simulink model "ModelCurrentState"  (R2024b)
settings: Solver=VariableStepAuto  StartTime=0.0  StopTime=StopTime  MaxStep=0.001  RelTol=1e-3
model workspace: external: MAT-File 3DModelInputs.mat (data not in the file)
undefined symbols (not defined in the file): GripStrength, KillswitchFinalValue, KillswitchInitialValue, KillswitchStepTime, LeftLowerArmLength, PlaneTilt, RightLowerArmLength, UpperTorsoLength, X, Y, Z
libraries: nesl_utility x408, sm_lib x139, matrix_library x11, simulink x1
(part 8 of 14)

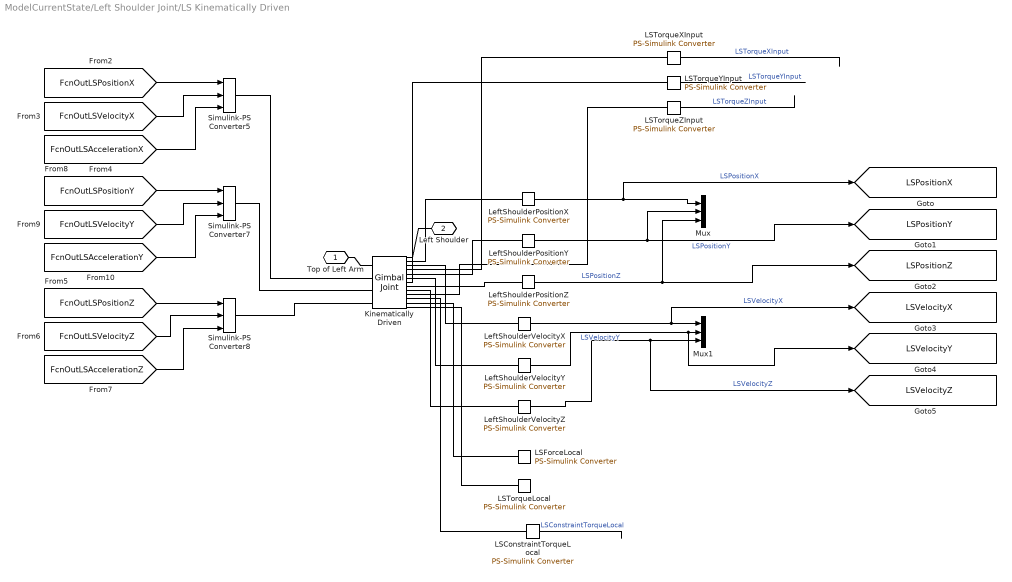
== system ModelCurrentState/Left Shoulder Joint/LS Kinematically Driven ==
  Kinematically Driven : sm_lib/Joints/Gimbal Joint  JointMode=Normal  CompositeWrenchDir=BaseOnFollower  CompositeWrenchFrame=FollowerFrame  SenseConstraintForce=off  SenseConstraintTorque=on  SenseTotalForce=on  SenseTotalTorque=on  RxPositionTargetSpecify=off  RxPositionTargetPriority=Low  RxPositionTargetValue=LSStartPositionX  RxPositionTargetValueUnits=deg  RxVelocityTargetSpecify=off  RxVelocityTargetPriority=Low  RxVelocityTargetValue=LSStartVelocityX  RxVelocityTargetValueUnits=deg/s  RxEquilibriumPosition=120  RxEquilibriumPositionUnits=deg  RxSpringStiffness=0  RxSpringStiffnessUnits=N*m/deg  RxDampingCoefficient=0  RxDampingCoefficientUnits=N*m/(deg/s)  RxLowerLimitSpecify=off  RxLowerLimitBound=-80  RxLowerLimitBoundUnits=deg  RxLowerLimitStiffness=100  RxLowerLimitStiffnessUnits=N*m/deg  RxLowerLimitDamping=10  RxLowerLimitDampingUnits=N*m/(deg/s)  RxLowerLimitTransitionRegionWidth=0.1  RxLowerLimitTransitionRegionWidthUnits=deg  RxUpperLimitSpecify=off  RxUpperLimitBound=80  RxUpperLimitBoundUnits=deg  RxUpperLimitStiffness=100  RxUpperLimitStiffnessUnits=N*m/deg  RxUpperLimitDamping=10  RxUpperLimitDampingUnits=N*m/(deg/s)  RxUpperLimitTransitionRegionWidth=0.1  RxUpperLimitTransitionRegionWidthUnits=deg  RxTorqueActuationMode=ComputedTorque  RxMotionActuationMode=InputMotion  RxSensePosition=on  RxSenseVelocity=on  RxSenseAcceleration=off  RxSenseTorqueForce=on  RxSenseLowerLimitTorqueForce=off  RxSenseUpperLimitTorqueForce=off  RyPositionTargetSpecify=off  RyPositionTargetPriority=Low  RyPositionTargetValue=LSStartPositionY  RyPositionTargetValueUnits=deg  RyVelocityTargetSpecify=off  RyVelocityTargetPriority=Low  RyVelocityTargetValue=LSStartVelocityY  RyVelocityTargetValueUnits=deg/s  RyEquilibriumPosition=0  RyEquilibriumPositionUnits=deg  RySpringStiffness=0  RySpringStiffnessUnits=N*m/deg  RyDampingCoefficient=0  RyDampingCoefficientUnits=N*m/(deg/s)  RyLowerLimitSpecify=off  RyLowerLimitBound=-80  RyLowerLimitBoundUnits=deg  RyLowerLimitStiffness=100  RyLowerLimitStiffnessUnits=N*m/deg  RyLowerLimitDamping=10  RyLowerLimitDampingUnits=N*m/(deg/s)  RyLowerLimitTransitionRegionWidth=0.1  RyLowerLimitTransitionRegionWidthUnits=deg  RyUpperLimitSpecify=off  RyUpperLimitBound=80  RyUpperLimitBoundUnits=deg  RyUpperLimitStiffness=100  RyUpperLimitStiffnessUnits=N*m/deg  RyUpperLimitDamping=10  RyUpperLimitDampingUnits=N*m/(deg/s)  RyUpperLimitTransitionRegionWidth=0.1  RyUpperLimitTransitionRegionWidthUnits=deg  RyTorqueActuationMode=ComputedTorque  RyMotionActuationMode=InputMotion  RySensePosition=on  RySenseVelocity=on  RySenseAcceleration=off  RySenseTorqueForce=on  RySenseLowerLimitTorqueForce=off  RySenseUpperLimitTorqueForce=off  RzPositionTargetSpecify=off  RzPositionTargetPriority=Low  RzPositionTargetValue=LSStartPositionZ  RzPositionTargetValueUnits=deg  RzVelocityTargetSpecify=off  RzVelocityTargetPriority=Low  RzVelocityTargetValue=LSStartVelocityZ  RzVelocityTargetValueUnits=deg/s  RzEquilibriumPosition=0  RzEquilibriumPositionUnits=deg  RzSpringStiffness=0  RzSpringStiffnessUnits=N*m/deg  RzDampingCoefficient=0  RzDampingCoefficientUnits=N*m/(deg/s)  RzLowerLimitSpecify=off  RzLowerLimitBound=-180  RzLowerLimitBoundUnits=deg  RzLowerLimitStiffness=100  RzLowerLimitStiffnessUnits=N*m/deg  RzLowerLimitDamping=10  RzLowerLimitDampingUnits=N*m/(deg/s)  RzLowerLimitTransitionRegionWidth=0.1  RzLowerLimitTransitionRegionWidthUnits=deg  RzUpperLimitSpecify=off  RzUpperLimitBound=-95  RzUpperLimitBoundUnits=deg  RzUpperLimitStiffness=100  RzUpperLimitStiffnessUnits=N*m/deg  RzUpperLimitDamping=10  RzUpperLimitDampingUnits=N*m/(deg/s)  RzUpperLimitTransitionRegionWidth=0.1  RzUpperLimitTransitionRegionWidthUnits=deg  RzTorqueActuationMode=ComputedTorque  RzMotionActuationMode=InputMotion  RzSensePosition=on  RzSenseVelocity=on  RzSenseAcceleration=off  RzSenseTorqueForce=on  RzSenseLowerLimitTorqueForce=off  RzSenseUpperLimitTorqueForce=off
  LSConstraintTorqueLocal : nesl_utility/PS-Simulink Converter  PhysicalDomain=network_engine_domain  SubClassName=ps_output  LeftPortType=input  RightPortType=output  PseudoPeriodic=off  Frequencies=[]  VectorFormat=1-D array  Unit=inherit  AffineConversion=off
  LSForceLocal : nesl_utility/PS-Simulink Converter  PhysicalDomain=network_engine_domain  SubClassName=ps_output  LeftPortType=input  RightPortType=output  PseudoPeriodic=off  Frequencies=[]  VectorFormat=1-D array  Unit=inherit  AffineConversion=off
  LSTorqueLocal : nesl_utility/PS-Simulink Converter  PhysicalDomain=network_engine_domain  SubClassName=ps_output  LeftPortType=input  RightPortType=output  PseudoPeriodic=off  Frequencies=[]  VectorFormat=1-D array  Unit=inherit  AffineConversion=off
  LSTorqueXInput : nesl_utility/PS-Simulink Converter  PhysicalDomain=network_engine_domain  SubClassName=ps_output  LeftPortType=input  RightPortType=output  PseudoPeriodic=off  Frequencies=[]  VectorFormat=1-D array  Unit=inherit  AffineConversion=off
  LSTorqueYInput : nesl_utility/PS-Simulink Converter  PhysicalDomain=network_engine_domain  SubClassName=ps_output  LeftPortType=input  RightPortType=output  PseudoPeriodic=off  Frequencies=[]  VectorFormat=1-D array  Unit=inherit  AffineConversion=off
  LSTorqueZInput : nesl_utility/PS-Simulink Converter  PhysicalDomain=network_engine_domain  SubClassName=ps_output  LeftPortType=input  RightPortType=output  PseudoPeriodic=off  Frequencies=[]  VectorFormat=1-D array  Unit=inherit  AffineConversion=off
  LeftShoulderPositionX : nesl_utility/PS-Simulink Converter  PhysicalDomain=network_engine_domain  SubClassName=ps_output  LeftPortType=input  RightPortType=output  PseudoPeriodic=off  Frequencies=[]  VectorFormat=1-D array  Unit=deg  AffineConversion=off
  LeftShoulderPositionY : nesl_utility/PS-Simulink Converter  PhysicalDomain=network_engine_domain  SubClassName=ps_output  LeftPortType=input  RightPortType=output  PseudoPeriodic=off  Frequencies=[]  VectorFormat=1-D array  Unit=deg  AffineConversion=off
  LeftShoulderPositionZ : nesl_utility/PS-Simulink Converter  PhysicalDomain=network_engine_domain  SubClassName=ps_output  LeftPortType=input  RightPortType=output  PseudoPeriodic=off  Frequencies=[]  VectorFormat=1-D array  Unit=deg  AffineConversion=off
  LeftShoulderVelocityX : nesl_utility/PS-Simulink Converter  PhysicalDomain=network_engine_domain  SubClassName=ps_output  LeftPortType=input  RightPortType=output  PseudoPeriodic=off  Frequencies=[]  VectorFormat=1-D array  Unit=deg/s  AffineConversion=off
  LeftShoulderVelocityY : nesl_utility/PS-Simulink Converter  PhysicalDomain=network_engine_domain  SubClassName=ps_output  LeftPortType=input  RightPortType=output  PseudoPeriodic=off  Frequencies=[]  VectorFormat=1-D array  Unit=deg/s  AffineConversion=off
  LeftShoulderVelocityZ : nesl_utility/PS-Simulink Converter  PhysicalDomain=network_engine_domain  SubClassName=ps_output  LeftPortType=input  RightPortType=output  PseudoPeriodic=off  Frequencies=[]  VectorFormat=1-D array  Unit=deg/s  AffineConversion=off
  Mux : Mux  Inputs=3
  Mux1 : Mux  Inputs=3
  Simulink-PS Converter5 : nesl_utility/Simulink-PS Converter  PhysicalDomain=network_engine_domain  SubClassName=ps_input  LeftPortType=input  RightPortType=output  PseudoPeriodic=off  Frequencies=[]  NoiseDistribution=none  NoiseParameters=[]  Unit=deg  AffineConversion=off  FilteringAndDerivatives=provide  SimscapeFilterOrder=1  InputFilterTimeConstant=0.001  UdotUserProvided=2
  Simulink-PS Converter7 : nesl_utility/Simulink-PS Converter  PhysicalDomain=network_engine_domain  SubClassName=ps_input  LeftPortType=input  RightPortType=output  PseudoPeriodic=off  Frequencies=[]  NoiseDistribution=none  NoiseParameters=[]  Unit=deg  AffineConversion=off  FilteringAndDerivatives=provide  SimscapeFilterOrder=1  InputFilterTimeConstant=0.001  UdotUserProvided=2
  Simulink-PS Converter8 : nesl_utility/Simulink-PS Converter  PhysicalDomain=network_engine_domain  SubClassName=ps_input  LeftPortType=input  RightPortType=output  PseudoPeriodic=off  Frequencies=[]  NoiseDistribution=none  NoiseParameters=[]  Unit=deg  AffineConversion=off  FilteringAndDerivatives=provide  SimscapeFilterOrder=1  InputFilterTimeConstant=0.001  UdotUserProvided=2
  Top of Left Arm : PMIOPort  Side=Left
  Left Shoulder : PMIOPort  Port=2  Side=Right
  tag scope: LSPositionX=global, LSPositionY=global, LSPositionZ=global, LSVelocityX=global, LSVelocityY=global, LSVelocityZ=global
  wires:
  [FcnOutLSPositionX] -> Simulink-PS Converter5/1
  [FcnOutLSPositionZ] -> Simulink-PS Converter8/1
  [FcnOutLSPositionY] -> Simulink-PS Converter7/1
  [FcnOutLSAccelerationZ] -> Simulink-PS Converter8/3
  [FcnOutLSAccelerationX] -> Simulink-PS Converter5/3
  [FcnOutLSAccelerationY] -> Simulink-PS Converter7/3
  [FcnOutLSVelocityY] -> Simulink-PS Converter7/2
  [FcnOutLSVelocityX] -> Simulink-PS Converter5/2
  [FcnOutLSVelocityZ] -> Simulink-PS Converter8/2
  LeftShoulderPositionY/1 -> [LSPositionY], Mux/2  "LSPositionY"
  LeftShoulderVelocityY/1 -> [LSVelocityY], Mux1/2  "LSVelocityY"
  LeftShoulderPositionZ/1 -> Mux/3, [LSPositionZ]  "LSPositionZ"
  LeftShoulderVelocityX/1 -> [LSVelocityX], Mux1/1  "LSVelocityX"
  LeftShoulderPositionX/1 -> [LSPositionX], Mux/1  "LSPositionX"
  LeftShoulderVelocityZ/1 -> [LSVelocityZ], Mux1/3  "LSVelocityZ"
  LSConstraintTorqueLocal/1 -> ?  "LSConstraintTorqueLocal"
  LSTorqueYInput/1 -> ?  "LSTorqueYInput"
  LSTorqueXInput/1 -> ?  "LSTorqueXInput"
  LSTorqueZInput/1 -> ?  "LSTorqueZInput"
  connections:
  Kinematically Driven/LConn1 -- Top of Left Arm/RConn1
  Simulink-PS Converter5/RConn1 -- Kinematically Driven/LConn2
  Simulink-PS Converter7/RConn1 -- Kinematically Driven/LConn3
  Simulink-PS Converter8/RConn1 -- Kinematically Driven/LConn4
  Left Shoulder/RConn1 -- Kinematically Driven/RConn1
  Kinematically Driven/RConn2 -- LeftShoulderPositionX/LConn1
  Kinematically Driven/RConn5 -- LeftShoulderPositionY/LConn1
  Kinematically Driven/RConn8 -- LeftShoulderPositionZ/LConn1
  Kinematically Driven/RConn3 -- LeftShoulderVelocityX/LConn1
  Kinematically Driven/RConn6 -- LeftShoulderVelocityY/LConn1
  Kinematically Driven/RConn9 -- LeftShoulderVelocityZ/LConn1
  LSForceLocal/LConn1 -- Kinematically Driven/RConn12
  LSTorqueLocal/LConn1 -- Kinematically Driven/RConn13
  Kinematically Driven/RConn11 -- LSConstraintTorqueLocal/LConn1
  LSTorqueXInput/LConn1 -- Kinematically Driven/RConn4
  LSTorqueYInput/LConn1 -- Kinematically Driven/RConn7
  LSTorqueZInput/LConn1 -- Kinematically Driven/RConn10

== system ModelCurrentState/Left Shoulder Joint/LS Kinetically Driven ==
  Kinetically Driven : sm_lib/Joints/Gimbal Joint  JointMode=Normal  CompositeWrenchDir=BaseOnFollower  CompositeWrenchFrame=FollowerFrame  SenseConstraintForce=off  SenseConstraintTorque=on  SenseTotalForce=on  SenseTotalTorque=on  RxPositionTargetSpecify=on  RxPositionTargetPriority=Low  RxPositionTargetValue=LSStartPositionX  RxPositionTargetValueUnits=deg  RxVelocityTargetSpecify=on  RxVelocityTargetPriority=Low  RxVelocityTargetValue=LSStartVelocityX  RxVelocityTargetValueUnits=deg/s  RxEquilibriumPosition=120  RxEquilibriumPositionUnits=deg  RxSpringStiffness=0  RxSpringStiffnessUnits=N*m/deg  RxDampingCoefficient=0  RxDampingCoefficientUnits=N*m/(deg/s)  RxLowerLimitSpecify=off  RxLowerLimitBound=-80  RxLowerLimitBoundUnits=deg  RxLowerLimitStiffness=100  RxLowerLimitStiffnessUnits=N*m/deg  RxLowerLimitDamping=10  RxLowerLimitDampingUnits=N*m/(deg/s)  RxLowerLimitTransitionRegionWidth=0.1  RxLowerLimitTransitionRegionWidthUnits=deg  RxUpperLimitSpecify=off  RxUpperLimitBound=80  RxUpperLimitBoundUnits=deg  RxUpperLimitStiffness=100  RxUpperLimitStiffnessUnits=N*m/deg  RxUpperLimitDamping=10  RxUpperLimitDampingUnits=N*m/(deg/s)  RxUpperLimitTransitionRegionWidth=0.1  RxUpperLimitTransitionRegionWidthUnits=deg  RxTorqueActuationMode=InputTorque  RxMotionActuationMode=ComputedMotion  RxSensePosition=on  RxSenseVelocity=on  RxSenseAcceleration=off  RxSenseTorqueForce=on  RxSenseLowerLimitTorqueForce=off  RxSenseUpperLimitTorqueForce=off  RyPositionTargetSpecify=on  RyPositionTargetPriority=Low  RyPositionTargetValue=LSStartPositionY  RyPositionTargetValueUnits=deg  RyVelocityTargetSpecify=on  RyVelocityTargetPriority=Low  RyVelocityTargetValue=LSStartVelocityY  RyVelocityTargetValueUnits=deg/s  RyEquilibriumPosition=0  RyEquilibriumPositionUnits=deg  RySpringStiffness=0  RySpringStiffnessUnits=N*m/deg  RyDampingCoefficient=0  RyDampingCoefficientUnits=N*m/(deg/s)  RyLowerLimitSpecify=off  RyLowerLimitBound=-80  RyLowerLimitBoundUnits=deg  RyLowerLimitStiffness=100  RyLowerLimitStiffnessUnits=N*m/deg  RyLowerLimitDamping=10  RyLowerLimitDampingUnits=N*m/(deg/s)  RyLowerLimitTransitionRegionWidth=0.1  RyLowerLimitTransitionRegionWidthUnits=deg  RyUpperLimitSpecify=off  RyUpperLimitBound=80  RyUpperLimitBoundUnits=deg  RyUpperLimitStiffness=100  RyUpperLimitStiffnessUnits=N*m/deg  RyUpperLimitDamping=10  RyUpperLimitDampingUnits=N*m/(deg/s)  RyUpperLimitTransitionRegionWidth=0.1  RyUpperLimitTransitionRegionWidthUnits=deg  RyTorqueActuationMode=InputTorque  RyMotionActuationMode=ComputedMotion  RySensePosition=on  RySenseVelocity=on  RySenseAcceleration=off  RySenseTorqueForce=on  RySenseLowerLimitTorqueForce=off  RySenseUpperLimitTorqueForce=off  RzPositionTargetSpecify=on  RzPositionTargetPriority=Low  RzPositionTargetValue=LSStartPositionZ  RzPositionTargetValueUnits=deg  RzVelocityTargetSpecify=on  RzVelocityTargetPriority=Low  RzVelocityTargetValue=LSStartVelocityZ  RzVelocityTargetValueUnits=deg/s  RzEquilibriumPosition=0  RzEquilibriumPositionUnits=deg  RzSpringStiffness=0  RzSpringStiffnessUnits=N*m/deg  RzDampingCoefficient=0  RzDampingCoefficientUnits=N*m/(deg/s)  RzLowerLimitSpecify=off  RzLowerLimitBound=-180  RzLowerLimitBoundUnits=deg  RzLowerLimitStiffness=100  RzLowerLimitStiffnessUnits=N*m/deg  RzLowerLimitDamping=10  RzLowerLimitDampingUnits=N*m/(deg/s)  RzLowerLimitTransitionRegionWidth=0.1  RzLowerLimitTransitionRegionWidthUnits=deg  RzUpperLimitSpecify=off  RzUpperLimitBound=-95  RzUpperLimitBoundUnits=deg  RzUpperLimitStiffness=100  RzUpperLimitStiffnessUnits=N*m/deg  RzUpperLimitDamping=10  RzUpperLimitDampingUnits=N*m/(deg/s)  RzUpperLimitTransitionRegionWidth=0.1  RzUpperLimitTransitionRegionWidthUnits=deg  RzTorqueActuationMode=InputTorque  RzMotionActuationMode=ComputedMotion  RzSensePosition=on  RzSenseVelocity=on  RzSenseAcceleration=off  RzSenseTorqueForce=on  RzSenseLowerLimitTorqueForce=off  RzSenseUpperLimitTorqueForce=off
  LSConstraintTorqueLocal : nesl_utility/PS-Simulink Converter  PhysicalDomain=network_engine_domain  SubClassName=ps_output  LeftPortType=input  RightPortType=output  PseudoPeriodic=off  Frequencies=[]  VectorFormat=1-D array  Unit=inherit  AffineConversion=off
  LSForceLocal : nesl_utility/PS-Simulink Converter  PhysicalDomain=network_engine_domain  SubClassName=ps_output  LeftPortType=input  RightPortType=output  PseudoPeriodic=off  Frequencies=[]  VectorFormat=1-D array  Unit=inherit  AffineConversion=off
  LSTorqueLocal : nesl_utility/PS-Simulink Converter  PhysicalDomain=network_engine_domain  SubClassName=ps_output  LeftPortType=input  RightPortType=output  PseudoPeriodic=off  Frequencies=[]  VectorFormat=1-D array  Unit=inherit  AffineConversion=off
  LSTorqueXInput : nesl_utility/PS-Simulink Converter  PhysicalDomain=network_engine_domain  SubClassName=ps_output  LeftPortType=input  RightPortType=output  PseudoPeriodic=off  Frequencies=[]  VectorFormat=1-D array  Unit=inherit  AffineConversion=off
  LSTorqueYInput : nesl_utility/PS-Simulink Converter  PhysicalDomain=network_engine_domain  SubClassName=ps_output  LeftPortType=input  RightPortType=output  PseudoPeriodic=off  Frequencies=[]  VectorFormat=1-D array  Unit=inherit  AffineConversion=off
  LSTorqueZInput : nesl_utility/PS-Simulink Converter  PhysicalDomain=network_engine_domain  SubClassName=ps_output  LeftPortType=input  RightPortType=output  PseudoPeriodic=off  Frequencies=[]  VectorFormat=1-D array  Unit=inherit  AffineConversion=off
  Left Shoulder Torque : nesl_utility/Simulink-PS Converter  PhysicalDomain=network_engine_domain  SubClassName=ps_input  LeftPortType=input  RightPortType=output  PseudoPeriodic=off  Frequencies=[]  NoiseDistribution=none  NoiseParameters=[]  Unit=N*m  AffineConversion=off  FilteringAndDerivatives=provide  SimscapeFilterOrder=1  InputFilterTimeConstant=0.001  UdotUserProvided=0
  LeftShoulderPositionX : nesl_utility/PS-Simulink Converter  PhysicalDomain=network_engine_domain  SubClassName=ps_output  LeftPortType=input  RightPortType=output  PseudoPeriodic=off  Frequencies=[]  VectorFormat=1-D array  Unit=deg  AffineConversion=off
  LeftShoulderPositionY : nesl_utility/PS-Simulink Converter  PhysicalDomain=network_engine_domain  SubClassName=ps_output  LeftPortType=input  RightPortType=output  PseudoPeriodic=off  Frequencies=[]  VectorFormat=1-D array  Unit=deg  AffineConversion=off
  LeftShoulderPositionZ : nesl_utility/PS-Simulink Converter  PhysicalDomain=network_engine_domain  SubClassName=ps_output  LeftPortType=input  RightPortType=output  PseudoPeriodic=off  Frequencies=[]  VectorFormat=1-D array  Unit=deg  AffineConversion=off
  LeftShoulderVelocityX : nesl_utility/PS-Simulink Converter  PhysicalDomain=network_engine_domain  SubClassName=ps_output  LeftPortType=input  RightPortType=output  PseudoPeriodic=off  Frequencies=[]  VectorFormat=1-D array  Unit=deg/s  AffineConversion=off
  LeftShoulderVelocityY : nesl_utility/PS-Simulink Converter  PhysicalDomain=network_engine_domain  SubClassName=ps_output  LeftPortType=input  RightPortType=output  PseudoPeriodic=off  Frequencies=[]  VectorFormat=1-D array  Unit=deg/s  AffineConversion=off
  LeftShoulderVelocityZ : nesl_utility/PS-Simulink Converter  PhysicalDomain=network_engine_domain  SubClassName=ps_output  LeftPortType=input  RightPortType=output  PseudoPeriodic=off  Frequencies=[]  VectorFormat=1-D array  Unit=deg/s  AffineConversion=off
  Mux : Mux  Inputs=3
  Mux1 : Mux  Inputs=3
  Simulink-PS Converter2 : nesl_utility/Simulink-PS Converter  PhysicalDomain=network_engine_domain  SubClassName=ps_input  LeftPortType=input  RightPortType=output  PseudoPeriodic=off  Frequencies=[]  NoiseDistribution=none  NoiseParameters=[]  Unit=1  AffineConversion=off  FilteringAndDerivatives=provide  SimscapeFilterOrder=1  InputFilterTimeConstant=0.001  UdotUserProvided=0
  Simulink-PS Converter6 : nesl_utility/Simulink-PS Converter  PhysicalDomain=network_engine_domain  SubClassName=ps_input  LeftPortType=input  RightPortType=output  PseudoPeriodic=off  Frequencies=[]  NoiseDistribution=none  NoiseParameters=[]  Unit=1  AffineConversion=off  FilteringAndDerivatives=provide  SimscapeFilterOrder=1  InputFilterTimeConstant=0.001  UdotUserProvided=0
  Top of Left Arm : PMIOPort  Side=Left
  Left Shoulder : PMIOPort  Port=2  Side=Right
  LSForceLocalOut : PMIOPort  Port=3  Side=Right
  LSTorqueLocalOut : PMIOPort  Port=4  Side=Right
  tag scope: LSPositionX=global, LSPositionY=global, LSPositionZ=global, LSVelocityX=global, LSVelocityY=global, LSVelocityZ=global
  wires:
  LeftShoulderVelocityZ/1 -> [LSVelocityZ], Mux1/3  "LSVelocityZ"
  [FcnOutLSTorqueZ] -> Left Shoulder Torque/1
  LeftShoulderPositionY/1 -> [LSPositionY], Mux/2  "LSPositionY"
  [FcnOutLSTorqueY] -> Simulink-PS Converter6/1
  LeftShoulderPositionZ/1 -> Mux/3, [LSPositionZ]  "LSPositionZ"
  LeftShoulderVelocityY/1 -> [LSVelocityY], Mux1/2  "LSVelocityY"
  LeftShoulderPositionX/1 -> [LSPositionX], Mux/1  "LSPositionX"
  LeftShoulderVelocityX/1 -> [LSVelocityX], Mux1/1  "LSVelocityX"
  [FcnOutLSTorqueX] -> Simulink-PS Converter2/1
  LSConstraintTorqueLocal/1 -> ?  "LSConstraintTorqueLocal"
  LSTorqueYInput/1 -> ?  "LSTorqueYInput"
  LSTorqueXInput/1 -> ?  "LSTorqueXInput"
  LSTorqueZInput/1 -> ?  "LSTorqueZInput"
  connections:
  Kinetically Driven/RConn3 -- LeftShoulderVelocityX/LConn1
  Simulink-PS Converter6/RConn1 -- Kinetically Driven/LConn3
  LSForceLocalOut/RConn1 -- LSForceLocal/LConn1 -- Kinetically Driven/RConn12
  LeftShoulderPositionX/LConn1 -- Kinetically Driven/RConn2
  Simulink-PS Converter2/RConn1 -- Kinetically Driven/LConn2
  LeftShoulderPositionZ/LConn1 -- Kinetically Driven/RConn8
  Left Shoulder Torque/RConn1 -- Kinetically Driven/LConn4
  LSTorqueLocalOut/RConn1 -- Kinetically Driven/RConn13 -- LSTorqueLocal/LConn1
  LeftShoulderVelocityY/LConn1 -- Kinetically Driven/RConn6
  LeftShoulderVelocityZ/LConn1 -- Kinetically Driven/RConn9
  Kinetically Driven/RConn5 -- LeftShoulderPositionY/LConn1
  Top of Left Arm/RConn1 -- Kinetically Driven/LConn1
  Left Shoulder/RConn1 -- Kinetically Driven/RConn1
  Kinetically Driven/RConn11 -- LSConstraintTorqueLocal/LConn1
  LSTorqueZInput/LConn1 -- Kinetically Driven/RConn10
  LSTorqueXInput/LConn1 -- Kinetically Driven/RConn4
  LSTorqueYInput/LConn1 -- Kinetically Driven/RConn7

== system ModelCurrentState/Left Upper Arm/Left Upper Arm MOF ==
  LElbowonLArmMOFLocal : Product  Multiplication=Matrix(*)
  LSAngularImpulseonArm : Integrator
  LShoulderonLArmMOFGlobal : matrix_library/Cross Product
  LShoulderonLArmMOFLocal : Product  Multiplication=Matrix(*)
  LUACOM : sm_lib/Body Elements/Inertia Sensor  SensorExtent=BodyGroup  SpanWeldJoints=off  ExcludeGroundedBodies=off  MeasurementFrame=World  SenseMass=off  SenseCenterOfMass=on  SenseInertiaMatrix=off  SenseCenteredInertiaMatrix=off  SensePrincipalInertiaMatrix=off  SenseRotationMatrix=off  GraphicType=None  PrincipalInertiaFrameSize=20  GraphicVisPropType=SimpleVisualProperties  GraphicDiffuseColor=[0.5 0.5 0.5]  GraphicOpacity=1  GraphicSpecularColor=[0.5 0.5 0.5 1.0]  GraphicAmbientColor=[0.15 0.15 0.15 1.0]  GraphicEmissiveColor=[0.0 0.0 0.0 1.0]  GraphicShininess=75
  Left Upper Arm COM : nesl_utility/PS-Simulink Converter  PhysicalDomain=network_engine_domain  SubClassName=ps_output  LeftPortType=input  RightPortType=output  PseudoPeriodic=off  Frequencies=[]  VectorFormat=1-D array  Unit=inherit  AffineConversion=off
  LeftElbowonLArmMOFGlobal : matrix_library/Cross Product
  R Vector Elbow Force on Left Arm : Sum  Inputs=-+
  R Vector Shoulder Force on Left Arm : Sum  Inputs=-+
  Rotation Transform Left Arm : nesl_utility/PS-Simulink Converter  PhysicalDomain=network_engine_domain  SubClassName=ps_output  LeftPortType=input  RightPortType=output  PseudoPeriodic=off  Frequencies=[]  VectorFormat=1-D array  Unit=inherit  AffineConversion=off
  SumofMomentsLArmLocal : Product  Multiplication=Matrix(*)
  SumofMomentsLSonLArm : Sum
  SumofMomentsLeftArmGlobal : Sum  Inputs=++++
  Transform Sensor : sm_lib/Frames and Transforms/Transform Sensor  MeasurementFrame=World  RotationSequence=XYX  SenseAngle=off  SenseAxis=off  SenseQ=off  SenseR=on  SenseRotationSequence=off  SenseOmegaX=off  SenseOmegaY=off  SenseOmegaZ=off  SenseOmega=off  SenseQDot=off  SenseRDot=off  SenseRotationSequenceDot=off  SenseAlphaX=off  SenseAlphaY=off  SenseAlphaZ=off  SenseAlpha=off  SenseQDDot=off  SenseRDDot=off  SenseX=off  SenseY=off  SenseZ=off  SenseXYZ=off  SenseRad=off  SenseAzim=off  SenseDist=off  SenseInc=off  SenseXDot=off  SenseYDot=off  SenseZDot=off  SenseXYZDot=off  SenseRadDot=off  SenseAzimDot=off  SenseDistDot=off  SenseIncDot=off  SenseXDDot=off  SenseYDDot=off  SenseZDDot=off  SenseXYZDDot=off  SenseRadDDot=off  SenseAzimDDot=off  SenseDistDDot=off  SenseIncDDot=off
  World Frame : sm_lib/Frames and Transforms/World Frame
  Left Upper Arm : PMIOPort  Side=Left
  wires:
  Left Upper Arm COM/1 -> R Vector Shoulder Force on Left Arm/1, R Vector Elbow Force on Left Arm/1  "LUpperArmCOM"
  [LEGlobalPosition] -> R Vector Elbow Force on Left Arm/2
  R Vector Elbow Force on Left Arm/1 -> LeftElbowonLArmMOFGlobal/1
  R Vector Shoulder Force on Left Arm/1 -> LShoulderonLArmMOFGlobal/1
  [LSGlobalPosition] -> R Vector Shoulder Force on Left Arm/2
  [LSonLArmFGlobalOut] -> LShoulderonLArmMOFGlobal/2
  [LForearmonLArmFGlobalOut] -> LeftElbowonLArmMOFGlobal/2
  [LForearmonLArmTGlobalOut] -> SumofMomentsLeftArmGlobal/4
  [LSonLArmTGlobalOut] -> SumofMomentsLSonLArm/1, SumofMomentsLeftArmGlobal/3
  Rotation Transform Left Arm/1 -> SumofMomentsLArmLocal/1, LElbowonLArmMOFLocal/1, LShoulderonLArmMOFLocal/1
  LShoulderonLArmMOFGlobal/1 -> SumofMomentsLeftArmGlobal/1, SumofMomentsLSonLArm/2, LShoulderonLArmMOFLocal/2  "LShoulderonLArmMOFGlobal"
  LeftElbowonLArmMOFGlobal/1 -> SumofMomentsLeftArmGlobal/2, LElbowonLArmMOFLocal/2  "LElbowonLArmMOFGlobal"
  SumofMomentsLeftArmGlobal/1 -> SumofMomentsLArmLocal/2  "SumofMomentsLeftArmGlobal"
  SumofMomentsLSonLArm/1 -> LSAngularImpulseonArm/1  "SumofMomentsLSonLArm"
  connections:
  LUACOM/LConn1 -- Transform Sensor/LConn1 -- Left Upper Arm/RConn1
  Left Upper Arm COM/LConn1 -- LUACOM/RConn1
  Transform Sensor/RConn1 -- World Frame/RConn1
  Rotation Transform Left Arm/LConn1 -- Transform Sensor/RConn2

== system ModelCurrentState/Left Wrist and Hand/LW Kinematically Driven ==
  LWConstraintTorqueLocal : nesl_utility/PS-Simulink Converter  PhysicalDomain=network_engine_domain  SubClassName=ps_output  LeftPortType=input  RightPortType=output  PseudoPeriodic=off  Frequencies=[]  VectorFormat=1-D array  Unit=inherit  AffineConversion=off
  LWForceLocal : nesl_utility/PS-Simulink Converter  PhysicalDomain=network_engine_domain  SubClassName=ps_output  LeftPortType=input  RightPortType=output  PseudoPeriodic=off  Frequencies=[]  VectorFormat=1-D array  Unit=inherit  AffineConversion=off
  LWTorqueLocal : nesl_utility/PS-Simulink Converter  PhysicalDomain=network_engine_domain  SubClassName=ps_output  LeftPortType=input  RightPortType=output  PseudoPeriodic=off  Frequencies=[]  VectorFormat=1-D array  Unit=inherit  AffineConversion=off
  LWTorqueXInput : nesl_utility/PS-Simulink Converter  PhysicalDomain=network_engine_domain  SubClassName=ps_output  LeftPortType=input  RightPortType=output  PseudoPeriodic=off  Frequencies=[]  VectorFormat=1-D array  Unit=inherit  AffineConversion=off
  LWTorqueYInput : nesl_utility/PS-Simulink Converter  PhysicalDomain=network_engine_domain  SubClassName=ps_output  LeftPortType=input  RightPortType=output  PseudoPeriodic=off  Frequencies=[]  VectorFormat=1-D array  Unit=inherit  AffineConversion=off
  Left Wrist Universal1 : sm_lib/Joints/Universal Joint  JointMode=Normal  CompositeWrenchDir=BaseOnFollower  CompositeWrenchFrame=FollowerFrame  SenseConstraintForce=off  SenseConstraintTorque=on  SenseTotalForce=on  SenseTotalTorque=on  RxPositionTargetSpecify=off  RxPositionTargetPriority=Low  RxPositionTargetValue=LWStartPositionX  RxPositionTargetValueUnits=deg  RxVelocityTargetSpecify=off  RxVelocityTargetPriority=Low  RxVelocityTargetValue=LWStartVelocityX  RxVelocityTargetValueUnits=deg/s  RxEquilibriumPosition=0  RxEquilibriumPositionUnits=deg  RxSpringStiffness=0  RxSpringStiffnessUnits=N*m/deg  RxDampingCoefficient=0  RxDampingCoefficientUnits=N*m/(deg/s)  RxLowerLimitSpecify=off  RxLowerLimitBound=-120  RxLowerLimitBoundUnits=deg  RxLowerLimitStiffness=300  RxLowerLimitStiffnessUnits=N*m/deg  RxLowerLimitDamping=10  RxLowerLimitDampingUnits=N*m/(deg/s)  RxLowerLimitTransitionRegionWidth=0.1  RxLowerLimitTransitionRegionWidthUnits=deg  RxUpperLimitSpecify=off  RxUpperLimitBound=0  RxUpperLimitBoundUnits=deg  RxUpperLimitStiffness=300  RxUpperLimitStiffnessUnits=N*m/deg  RxUpperLimitDamping=10  RxUpperLimitDampingUnits=N*m/(deg/s)  RxUpperLimitTransitionRegionWidth=0.1  RxUpperLimitTransitionRegionWidthUnits=deg  RxTorqueActuationMode=ComputedTorque  RxMotionActuationMode=InputMotion  RxSensePosition=on  RxSenseVelocity=on  RxSenseAcceleration=off  RxSenseTorqueForce=on  RxSenseLowerLimitTorqueForce=off  RxSenseUpperLimitTorqueForce=off  RyPositionTargetSpecify=off  RyPositionTargetPriority=Low  RyPositionTargetValue=LWStartPositionY  RyPositionTargetValueUnits=deg  RyVelocityTargetSpecify=off  RyVelocityTargetPriority=Low  RyVelocityTargetValue=LWStartVelocityY  RyVelocityTargetValueUnits=deg/s  RyEquilibriumPosition=0  RyEquilibriumPositionUnits=deg  RySpringStiffness=0  RySpringStiffnessUnits=N*m/deg  RyDampingCoefficient=0  RyDampingCoefficientUnits=N*m/(deg/s)  RyLowerLimitSpecify=off  RyLowerLimitBound=-30  RyLowerLimitBoundUnits=deg  RyLowerLimitStiffness=300  RyLowerLimitStiffnessUnits=N*m/deg  RyLowerLimitDamping=10  RyLowerLimitDampingUnits=N*m/(deg/s)  RyLowerLimitTransitionRegionWidth=0.1  RyLowerLimitTransitionRegionWidthUnits=deg  RyUpperLimitSpecify=off  RyUpperLimitBound=30  RyUpperLimitBoundUnits=deg  RyUpperLimitStiffness=300  RyUpperLimitStiffnessUnits=N*m/deg  RyUpperLimitDamping=10  RyUpperLimitDampingUnits=N*m/(deg/s)  RyUpperLimitTransitionRegionWidth=0.1  RyUpperLimitTransitionRegionWidthUnits=deg  RyTorqueActuationMode=ComputedTorque  RyMotionActuationMode=InputMotion  RySensePosition=on  RySenseVelocity=on  RySenseAcceleration=off  RySenseTorqueForce=on  RySenseLowerLimitTorqueForce=off  RySenseUpperLimitTorqueForce=off
  LeftWristPositionX : nesl_utility/PS-Simulink Converter  PhysicalDomain=network_engine_domain  SubClassName=ps_output  LeftPortType=input  RightPortType=output  PseudoPeriodic=off  Frequencies=[]  VectorFormat=1-D array  Unit=deg  AffineConversion=off
  LeftWristPositionY : nesl_utility/PS-Simulink Converter  PhysicalDomain=network_engine_domain  SubClassName=ps_output  LeftPortType=input  RightPortType=output  PseudoPeriodic=off  Frequencies=[]  VectorFormat=1-D array  Unit=deg  AffineConversion=off
  LeftWristVelocityX : nesl_utility/PS-Simulink Converter  PhysicalDomain=network_engine_domain  SubClassName=ps_output  LeftPortType=input  RightPortType=output  PseudoPeriodic=off  Frequencies=[]  VectorFormat=1-D array  Unit=deg/s  AffineConversion=off
  LeftWristVelocityY : nesl_utility/PS-Simulink Converter  PhysicalDomain=network_engine_domain  SubClassName=ps_output  LeftPortType=input  RightPortType=output  PseudoPeriodic=off  Frequencies=[]  VectorFormat=1-D array  Unit=deg/s  AffineConversion=off
  Simulink-PS Converter24 : nesl_utility/Simulink-PS Converter  PhysicalDomain=network_engine_domain  SubClassName=ps_input  LeftPortType=input  RightPortType=output  PseudoPeriodic=off  Frequencies=[]  NoiseDistribution=none  NoiseParameters=[]  Unit=deg  AffineConversion=off  FilteringAndDerivatives=provide  SimscapeFilterOrder=1  InputFilterTimeConstant=0.001  UdotUserProvided=2
  Simulink-PS Converter26 : nesl_utility/Simulink-PS Converter  PhysicalDomain=network_engine_domain  SubClassName=ps_input  LeftPortType=input  RightPortType=output  PseudoPeriodic=off  Frequencies=[]  NoiseDistribution=none  NoiseParameters=[]  Unit=deg  AffineConversion=off  FilteringAndDerivatives=provide  SimscapeFilterOrder=1  InputFilterTimeConstant=0.001  UdotUserProvided=2
  Subtract : Sum  Inputs=+-
  LH Grip Standoff : PMIOPort  Side=Right
  LW : PMIOPort  Port=2  Side=Left
  tag scope: LWConstraintTorqueLocal=global, LWForceLocal=global, LWPositionX=global, LWPositionY=global, LWTorqueLocal=global, LWTotalMinusConstraintTorque=global, LWVelocityX=global, LWVelocityY=global
  wires:
  [FcnOutLWVelocityY] -> Simulink-PS Converter26/2
  [FcnOutLWAccelerationX] -> Simulink-PS Converter24/3
  [FcnOutLWAccelerationY] -> Simulink-PS Converter26/3
  [FcnOutLWPositionY] -> Simulink-PS Converter26/1
  [FcnOutLWVelocityX] -> Simulink-PS Converter24/2
  [FcnOutLWPositionX] -> Simulink-PS Converter24/1
  LeftWristVelocityY/1 -> [LWVelocityY]  "LWVelocityY"
  LeftWristVelocityX/1 -> [LWVelocityX]  "LWVelocityX"
  LeftWristPositionX/1 -> [LWPositionX]  "LWPositionX"
  LeftWristPositionY/1 -> [LWPositionY]  "LWPositionY"
  LWForceLocal/1 -> [LWForceLocal]  "LWForceLocal"
  Subtract/1 -> [LWTotalMinusConstraintTorque]  "LWTotalMinusConstraintTorque"
  LWConstraintTorqueLocal/1 -> Subtract/2, [LWConstraintTorqueLocal]  "LWConstraintTorqueLocal"
  LWTorqueLocal/1 -> Subtract/1, [LWTorqueLocal]  "LWTorqueLocal"
  LWTorqueXInput/1 -> ?  "LWTorqueXInput"
  LWTorqueYInput/1 -> ?  "LWTorqueYInput"
  connections:
  Left Wrist Universal1/LConn3 -- Simulink-PS Converter26/RConn1
  Left Wrist Universal1/LConn2 -- Simulink-PS Converter24/RConn1
  Left Wrist Universal1/LConn1 -- LW/RConn1
  Left Wrist Universal1/RConn1 -- LH Grip Standoff/RConn1
  Left Wrist Universal1/RConn2 -- LeftWristPositionX/LConn1
  Left Wrist Universal1/RConn3 -- LeftWristVelocityX/LConn1
  Left Wrist Universal1/RConn5 -- LeftWristPositionY/LConn1
  Left Wrist Universal1/RConn6 -- LeftWristVelocityY/LConn1
  LWForceLocal/LConn1 -- Left Wrist Universal1/RConn9
  LWTorqueLocal/LConn1 -- Left Wrist Universal1/RConn10
  Left Wrist Universal1/RConn8 -- LWConstraintTorqueLocal/LConn1
  LWTorqueYInput/LConn1 -- Left Wrist Universal1/RConn7
  LWTorqueXInput/LConn1 -- Left Wrist Universal1/RConn4

== system ModelCurrentState/Left Wrist and Hand/LW Kinetically Driven ==
  LWConstraintTorqueLocal : nesl_utility/PS-Simulink Converter  PhysicalDomain=network_engine_domain  SubClassName=ps_output  LeftPortType=input  RightPortType=output  PseudoPeriodic=off  Frequencies=[]  VectorFormat=1-D array  Unit=inherit  AffineConversion=off
  LWForceLocal : nesl_utility/PS-Simulink Converter  PhysicalDomain=network_engine_domain  SubClassName=ps_output  LeftPortType=input  RightPortType=output  PseudoPeriodic=off  Frequencies=[]  VectorFormat=1-D array  Unit=inherit  AffineConversion=off
  LWTorqueLocal : nesl_utility/PS-Simulink Converter  PhysicalDomain=network_engine_domain  SubClassName=ps_output  LeftPortType=input  RightPortType=output  PseudoPeriodic=off  Frequencies=[]  VectorFormat=1-D array  Unit=inherit  AffineConversion=off
  LWTorqueXInput : nesl_utility/PS-Simulink Converter  PhysicalDomain=network_engine_domain  SubClassName=ps_output  LeftPortType=input  RightPortType=output  PseudoPeriodic=off  Frequencies=[]  VectorFormat=1-D array  Unit=inherit  AffineConversion=off
  LWTorqueYInput : nesl_utility/PS-Simulink Converter  PhysicalDomain=network_engine_domain  SubClassName=ps_output  LeftPortType=input  RightPortType=output  PseudoPeriodic=off  Frequencies=[]  VectorFormat=1-D array  Unit=inherit  AffineConversion=off
  Left Wrist TX : nesl_utility/Simulink-PS Converter  PhysicalDomain=network_engine_domain  SubClassName=ps_input  LeftPortType=input  RightPortType=output  PseudoPeriodic=off  Frequencies=[]  NoiseDistribution=none  NoiseParameters=[]  Unit=N*m  AffineConversion=off  FilteringAndDerivatives=provide  SimscapeFilterOrder=1  InputFilterTimeConstant=0.001  UdotUserProvided=0
  Left Wrist TY : nesl_utility/Simulink-PS Converter  PhysicalDomain=network_engine_domain  SubClassName=ps_input  LeftPortType=input  RightPortType=output  PseudoPeriodic=off  Frequencies=[]  NoiseDistribution=none  NoiseParameters=[]  Unit=N*m  AffineConversion=off  FilteringAndDerivatives=provide  SimscapeFilterOrder=1  InputFilterTimeConstant=0.001  UdotUserProvided=0
  Left Wrist Universal : sm_lib/Joints/Universal Joint  JointMode=Normal  CompositeWrenchDir=BaseOnFollower  CompositeWrenchFrame=FollowerFrame  SenseConstraintForce=off  SenseConstraintTorque=on  SenseTotalForce=on  SenseTotalTorque=on  RxPositionTargetSpecify=on  RxPositionTargetPriority=Low  RxPositionTargetValue=LWStartPositionX  RxPositionTargetValueUnits=deg  RxVelocityTargetSpecify=on  RxVelocityTargetPriority=Low  RxVelocityTargetValue=LWStartVelocityX  RxVelocityTargetValueUnits=deg/s  RxEquilibriumPosition=0  RxEquilibriumPositionUnits=deg  RxSpringStiffness=0  RxSpringStiffnessUnits=N*m/deg  RxDampingCoefficient=0  RxDampingCoefficientUnits=N*m/(deg/s)  RxLowerLimitSpecify=off  RxLowerLimitBound=-120  RxLowerLimitBoundUnits=deg  RxLowerLimitStiffness=300  RxLowerLimitStiffnessUnits=N*m/deg  RxLowerLimitDamping=10  RxLowerLimitDampingUnits=N*m/(deg/s)  RxLowerLimitTransitionRegionWidth=0.1  RxLowerLimitTransitionRegionWidthUnits=deg  RxUpperLimitSpecify=off  RxUpperLimitBound=0  RxUpperLimitBoundUnits=deg  RxUpperLimitStiffness=300  RxUpperLimitStiffnessUnits=N*m/deg  RxUpperLimitDamping=10  RxUpperLimitDampingUnits=N*m/(deg/s)  RxUpperLimitTransitionRegionWidth=0.1  RxUpperLimitTransitionRegionWidthUnits=deg  RxTorqueActuationMode=InputTorque  RxMotionActuationMode=ComputedMotion  RxSensePosition=on  RxSenseVelocity=on  RxSenseAcceleration=off  RxSenseTorqueForce=on  RxSenseLowerLimitTorqueForce=off  RxSenseUpperLimitTorqueForce=off  RyPositionTargetSpecify=on  RyPositionTargetPriority=Low  RyPositionTargetValue=LWStartPositionY  RyPositionTargetValueUnits=deg  RyVelocityTargetSpecify=on  RyVelocityTargetPriority=Low  RyVelocityTargetValue=LWStartVelocityY  RyVelocityTargetValueUnits=deg/s  RyEquilibriumPosition=0  RyEquilibriumPositionUnits=deg  RySpringStiffness=0  RySpringStiffnessUnits=N*m/deg  RyDampingCoefficient=0  RyDampingCoefficientUnits=N*m/(deg/s)  RyLowerLimitSpecify=off  RyLowerLimitBound=-30  RyLowerLimitBoundUnits=deg  RyLowerLimitStiffness=300  RyLowerLimitStiffnessUnits=N*m/deg  RyLowerLimitDamping=10  RyLowerLimitDampingUnits=N*m/(deg/s)  RyLowerLimitTransitionRegionWidth=0.1  RyLowerLimitTransitionRegionWidthUnits=deg  RyUpperLimitSpecify=off  RyUpperLimitBound=30  RyUpperLimitBoundUnits=deg  RyUpperLimitStiffness=300  RyUpperLimitStiffnessUnits=N*m/deg  RyUpperLimitDamping=10  RyUpperLimitDampingUnits=N*m/(deg/s)  RyUpperLimitTransitionRegionWidth=0.1  RyUpperLimitTransitionRegionWidthUnits=deg  RyTorqueActuationMode=InputTorque  RyMotionActuationMode=ComputedMotion  RySensePosition=on  RySenseVelocity=on  RySenseAcceleration=off  RySenseTorqueForce=on  RySenseLowerLimitTorqueForce=off  RySenseUpperLimitTorqueForce=off
  LeftWristPositionX : nesl_utility/PS-Simulink Converter  PhysicalDomain=network_engine_domain  SubClassName=ps_output  LeftPortType=input  RightPortType=output  PseudoPeriodic=off  Frequencies=[]  VectorFormat=1-D array  Unit=deg  AffineConversion=off
  LeftWristPositionY : nesl_utility/PS-Simulink Converter  PhysicalDomain=network_engine_domain  SubClassName=ps_output  LeftPortType=input  RightPortType=output  PseudoPeriodic=off  Frequencies=[]  VectorFormat=1-D array  Unit=deg  AffineConversion=off
  LeftWristVelocityX : nesl_utility/PS-Simulink Converter  PhysicalDomain=network_engine_domain  SubClassName=ps_output  LeftPortType=input  RightPortType=output  PseudoPeriodic=off  Frequencies=[]  VectorFormat=1-D array  Unit=deg/s  AffineConversion=off
  LeftWristVelocityY : nesl_utility/PS-Simulink Converter  PhysicalDomain=network_engine_domain  SubClassName=ps_output  LeftPortType=input  RightPortType=output  PseudoPeriodic=off  Frequencies=[]  VectorFormat=1-D array  Unit=deg/s  AffineConversion=off
  Subtract : Sum  Inputs=+-
  LW : PMIOPort  Side=Left
  LH Grip Standoff : PMIOPort  Port=2  Side=Right
  tag scope: LWConstraintTorqueLocal=global, LWForceLocal=global, LWPositionX=global, LWPositionY=global, LWTorqueLocal=global, LWTotalMinusConstraintTorque=global, LWVelocityX=global, LWVelocityY=global
  wires:
  [FcnOutLWTorqueY] -> Left Wrist TY/1
  LeftWristPositionX/1 -> [LWPositionX]  "LWPositionX"
  LeftWristPositionY/1 -> [LWPositionY]  "LWPositionY"
  [FcnOutLWTorqueX] -> Left Wrist TX/1
  LeftWristVelocityX/1 -> [LWVelocityX]  "LWVelocityX"
  LeftWristVelocityY/1 -> [LWVelocityY]  "LWVelocityY"
  LWForceLocal/1 -> [LWForceLocal]  "LWForceLocal"
  LWTorqueLocal/1 -> Subtract/1, [LWTorqueLocal]  "LWTorqueLocal"
  LWConstraintTorqueLocal/1 -> [LWConstraintTorqueLocal], Subtract/2  "LWConstraintTorqueLocal"
  Subtract/1 -> [LWTotalMinusConstraintTorque]  "LWTotalMinusConstraintTorque"
  LWTorqueXInput/1 -> ?  "LWTorqueXInput"
  LWTorqueYInput/1 -> ?  "LWTorqueYInput"
  connections:
  Left Wrist Universal/LConn1 -- LW/RConn1
  Left Wrist Universal/RConn9 -- LWForceLocal/LConn1
  Left Wrist Universal/LConn2 -- Left Wrist TX/RConn1
  Left Wrist Universal/RConn5 -- LeftWristPositionY/LConn1
  Left Wrist Universal/RConn6 -- LeftWristVelocityY/LConn1
  Left Wrist Universal/LConn3 -- Left Wrist TY/RConn1
  Left Wrist Universal/RConn2 -- LeftWristPositionX/LConn1
  Left Wrist Universal/RConn3 -- LeftWristVelocityX/LConn1
  Left Wrist Universal/RConn10 -- LWTorqueLocal/LConn1
  Left Wrist Universal/RConn1 -- LH Grip Standoff/RConn1
  LWConstraintTorqueLocal/LConn1 -- Left Wrist Universal/RConn8
  LWTorqueXInput/LConn1 -- Left Wrist Universal/RConn4
  Left Wrist Universal/RConn7 -- LWTorqueYInput/LConn1

== system ModelCurrentState/Right Elbow Joint/RE Kinematically Driven ==
  Kinematically Driven RE : sm_lib/Joints/Revolute Joint  JointMode=Normal  CompositeWrenchDir=BaseOnFollower  CompositeWrenchFrame=FollowerFrame  SenseConstraintForce=off  SenseConstraintTorque=on  SenseTotalForce=on  SenseTotalTorque=on  PositionTargetSpecify=off  PositionTargetPriority=Low  PositionTargetValue=REStartPosition  PositionTargetValueUnits=deg  VelocityTargetSpecify=off  VelocityTargetPriority=Low  VelocityTargetValue=REStartVelocity  VelocityTargetValueUnits=deg/s  EquilibriumPosition=0  EquilibriumPositionUnits=deg  SpringStiffness=0  SpringStiffnessUnits=N*m/deg  DampingCoefficient=0  DampingCoefficientUnits=N*m/(deg/s)  LowerLimitSpecify=off  LowerLimitBound=0  LowerLimitBoundUnits=deg  LowerLimitStiffness=20  LowerLimitStiffnessUnits=N*m/deg  LowerLimitDamping=0  LowerLimitDampingUnits=N*m/(deg/s)  LowerLimitTransitionRegionWidth=0.1  LowerLimitTransitionRegionWidthUnits=deg  UpperLimitSpecify=off  UpperLimitBound=120  UpperLimitBoundUnits=deg  UpperLimitStiffness=100  UpperLimitStiffnessUnits=N*m/deg  UpperLimitDamping=0  UpperLimitDampingUnits=N*m/(deg/s)  UpperLimitTransitionRegionWidth=0.1  UpperLimitTransitionRegionWidthUnits=deg  TorqueActuationMode=ComputedTorque  MotionActuationMode=InputMotion  SensePosition=on  SenseVelocity=on  SenseAcceleration=off  SenseTorqueForce=on  SenseLowerLimitTorqueForce=off  SenseUpperLimitTorqueForce=off
      settings: LogSimulationData=on
  REConstraintTorqueLocal : nesl_utility/PS-Simulink Converter  PhysicalDomain=network_engine_domain  SubClassName=ps_output  LeftPortType=input  RightPortType=output  PseudoPeriodic=off  Frequencies=[]  VectorFormat=1-D array  Unit=inherit  AffineConversion=off
  REForceLocal : nesl_utility/PS-Simulink Converter  PhysicalDomain=network_engine_domain  SubClassName=ps_output  LeftPortType=input  RightPortType=output  PseudoPeriodic=off  Frequencies=[]  VectorFormat=1-D array  Unit=inherit  AffineConversion=off
  RETorqueInput : nesl_utility/PS-Simulink Converter  PhysicalDomain=network_engine_domain  SubClassName=ps_output  LeftPortType=input  RightPortType=output  PseudoPeriodic=off  Frequencies=[]  VectorFormat=1-D array  Unit=inherit  AffineConversion=off
  RETorqueLocal : nesl_utility/PS-Simulink Converter  PhysicalDomain=network_engine_domain  SubClassName=ps_output  LeftPortType=input  RightPortType=output  PseudoPeriodic=off  Frequencies=[]  VectorFormat=1-D array  Unit=inherit  AffineConversion=off
  RightElbowPosition : nesl_utility/PS-Simulink Converter  PhysicalDomain=network_engine_domain  SubClassName=ps_output  LeftPortType=input  RightPortType=output  PseudoPeriodic=off  Frequencies=[]  VectorFormat=1-D array  Unit=deg  AffineConversion=off
  RightElbowVelocity : nesl_utility/PS-Simulink Converter  PhysicalDomain=network_engine_domain  SubClassName=ps_output  LeftPortType=input  RightPortType=output  PseudoPeriodic=off  Frequencies=[]  VectorFormat=1-D array  Unit=deg/s  AffineConversion=off
  Simulink-PS Converter29 : nesl_utility/Simulink-PS Converter  PhysicalDomain=network_engine_domain  SubClassName=ps_input  LeftPortType=input  RightPortType=output  PseudoPeriodic=off  Frequencies=[]  NoiseDistribution=none  NoiseParameters=[]  Unit=deg  AffineConversion=off  FilteringAndDerivatives=provide  SimscapeFilterOrder=1  InputFilterTimeConstant=0.001  UdotUserProvided=2
  Bottom of Right Arm : PMIOPort  Side=Left
  Top of Right Forearm : PMIOPort  Port=2  Side=Right
  tag scope: REPosition=global, REVelocity=global
  wires:
  [FcnOutREVelocity] -> Simulink-PS Converter29/2
  [FcnOutREAcceleration] -> Simulink-PS Converter29/3
  [FcnOutREPosition] -> Simulink-PS Converter29/1
  RightElbowVelocity/1 -> [REVelocity]  "REVelocity"
  RightElbowPosition/1 -> [REPosition]  "REPosition"
  REConstraintTorqueLocal/1 -> ?  "REConstraintTorqueLocal"
  RETorqueInput/1 -> ?  "RETorqueInput"
  connections:
  Kinematically Driven RE/LConn1 -- Bottom of Right Arm/RConn1
  Simulink-PS Converter29/RConn1 -- Kinematically Driven RE/LConn2
  Kinematically Driven RE/RConn1 -- Top of Right Forearm/RConn1
  RETorqueLocal/LConn1 -- Kinematically Driven RE/RConn7
  REForceLocal/LConn1 -- Kinematically Driven RE/RConn6
  RightElbowPosition/LConn1 -- Kinematically Driven RE/RConn2
  RightElbowVelocity/LConn1 -- Kinematically Driven RE/RConn3
  Kinematically Driven RE/RConn5 -- REConstraintTorqueLocal/LConn1
  RETorqueInput/LConn1 -- Kinematically Driven RE/RConn4

== system ModelCurrentState/Right Elbow Joint/RE Kinetically Driven ==
  Kinetically Driven RE : sm_lib/Joints/Revolute Joint  JointMode=Normal  CompositeWrenchDir=BaseOnFollower  CompositeWrenchFrame=FollowerFrame  SenseConstraintForce=off  SenseConstraintTorque=on  SenseTotalForce=on  SenseTotalTorque=on  PositionTargetSpecify=on  PositionTargetPriority=Low  PositionTargetValue=REStartPosition  PositionTargetValueUnits=deg  VelocityTargetSpecify=off  VelocityTargetPriority=Low  VelocityTargetValue=REStartVelocity  VelocityTargetValueUnits=deg/s  EquilibriumPosition=0  EquilibriumPositionUnits=deg  SpringStiffness=0  SpringStiffnessUnits=N*m/deg  DampingCoefficient=0  DampingCoefficientUnits=N*m/(deg/s)  LowerLimitSpecify=off  LowerLimitBound=0  LowerLimitBoundUnits=deg  LowerLimitStiffness=20  LowerLimitStiffnessUnits=N*m/deg  LowerLimitDamping=0  LowerLimitDampingUnits=N*m/(deg/s)  LowerLimitTransitionRegionWidth=0.1  LowerLimitTransitionRegionWidthUnits=deg  UpperLimitSpecify=off  UpperLimitBound=120  UpperLimitBoundUnits=deg  UpperLimitStiffness=100  UpperLimitStiffnessUnits=N*m/deg  UpperLimitDamping=0  UpperLimitDampingUnits=N*m/(deg/s)  UpperLimitTransitionRegionWidth=0.1  UpperLimitTransitionRegionWidthUnits=deg  TorqueActuationMode=InputTorque  MotionActuationMode=ComputedMotion  SensePosition=on  SenseVelocity=on  SenseAcceleration=off  SenseTorqueForce=on  SenseLowerLimitTorqueForce=off  SenseUpperLimitTorqueForce=off
      settings: LogSimulationData=on
  REConstraintTorqueLocal : nesl_utility/PS-Simulink Converter  PhysicalDomain=network_engine_domain  SubClassName=ps_output  LeftPortType=input  RightPortType=output  PseudoPeriodic=off  Frequencies=[]  VectorFormat=1-D array  Unit=inherit  AffineConversion=off
  REForceLocal : nesl_utility/PS-Simulink Converter  PhysicalDomain=network_engine_domain  SubClassName=ps_output  LeftPortType=input  RightPortType=output  PseudoPeriodic=off  Frequencies=[]  VectorFormat=1-D array  Unit=inherit  AffineConversion=off
  RETorqueInput : nesl_utility/PS-Simulink Converter  PhysicalDomain=network_engine_domain  SubClassName=ps_output  LeftPortType=input  RightPortType=output  PseudoPeriodic=off  Frequencies=[]  VectorFormat=1-D array  Unit=inherit  AffineConversion=off
  RETorqueLocal : nesl_utility/PS-Simulink Converter  PhysicalDomain=network_engine_domain  SubClassName=ps_output  LeftPortType=input  RightPortType=output  PseudoPeriodic=off  Frequencies=[]  VectorFormat=1-D array  Unit=inherit  AffineConversion=off
  Right Elbow Torque1 : nesl_utility/Simulink-PS Converter  PhysicalDomain=network_engine_domain  SubClassName=ps_input  LeftPortType=input  RightPortType=output  PseudoPeriodic=off  Frequencies=[]  NoiseDistribution=none  NoiseParameters=[]  Unit=N*m  AffineConversion=off  FilteringAndDerivatives=provide  SimscapeFilterOrder=1  InputFilterTimeConstant=0.001  UdotUserProvided=0
  RightElbowPosition : nesl_utility/PS-Simulink Converter  PhysicalDomain=network_engine_domain  SubClassName=ps_output  LeftPortType=input  RightPortType=output  PseudoPeriodic=off  Frequencies=[]  VectorFormat=1-D array  Unit=deg  AffineConversion=off
  RightElbowVelocity : nesl_utility/PS-Simulink Converter  PhysicalDomain=network_engine_domain  SubClassName=ps_output  LeftPortType=input  RightPortType=output  PseudoPeriodic=off  Frequencies=[]  VectorFormat=1-D array  Unit=deg/s  AffineConversion=off
  Bottom of Right Arm : PMIOPort  Side=Left
  RE Force Local Out : PMIOPort  Port=2  Side=Right
  RE Torque Local Out : PMIOPort  Port=3  Side=Right
  Top of Right Forearm : PMIOPort  Port=4  Side=Right
  tag scope: REPosition=global, REVelocity=global
  wires:
  RightElbowPosition/1 -> [REPosition]  "REPosition"
  [FcnOutRETorque] -> Right Elbow Torque1/1
  RightElbowVelocity/1 -> [REVelocity]  "REVelocity"
  REConstraintTorqueLocal/1 -> ?  "REConstraintTorqueLocal"
  RETorqueInput/1 -> ?  "RETorqueInput"
  connections:
  Kinetically Driven RE/RConn3 -- RightElbowVelocity/LConn1
  Kinetically Driven RE/RConn2 -- RightElbowPosition/LConn1
  RE Force Local Out/RConn1 -- Kinetically Driven RE/RConn6 -- REForceLocal/LConn1
  Right Elbow Torque1/RConn1 -- Kinetically Driven RE/LConn2
  RE Torque Local Out/RConn1 -- Kinetically Driven RE/RConn7 -- RETorqueLocal/LConn1
  Bottom of Right Arm/RConn1 -- Kinetically Driven RE/LConn1
  Top of Right Forearm/RConn1 -- Kinetically Driven RE/RConn1
  REConstraintTorqueLocal/LConn1 -- Kinetically Driven RE/RConn5
  RETorqueInput/LConn1 -- Kinetically Driven RE/RConn4
